simulink model "PlantModelSim"  (R2019b)
settings: Solver=VariableStepAuto  StartTime=0.0  StopTime=10.0  RelTol=1e-3
values from neighbouring files (symbols this model uses):
  A = [0  0  0  1  0  0  0  0  0  0  0  0 ... (first row only)    [Naman_LQR_Working.m]    (also in PlantModel.m = [0  0  0  1  0  0  0  0  0  0  0  0;      0  0  0  0  1  0  )
  B = [0      0       0       0 ... (first row only)    [Naman_LQR_Working.m]    (also in PlantModel.m = [0 0 0 0;      0 0 0 0;      0 0 0 0;      0 0 0 0;      0 0)
  C = [1 0 0 0 0 0 0 0 0 0 0 0 ... (first row only)    [Naman_LQR_Working.m]    (also in PlantModel.m = [1 0 0 0 0 0 0 0 0 0 0 0;      0 1 0 0 0 0 0 0 0 0 0 0;     )
  D = zeros(6,4)    [Naman_LQR_Working.m]    (also in PlantModel.m)
settings Model: Creator=Lakshu  LastModifiedBy=Lakshu

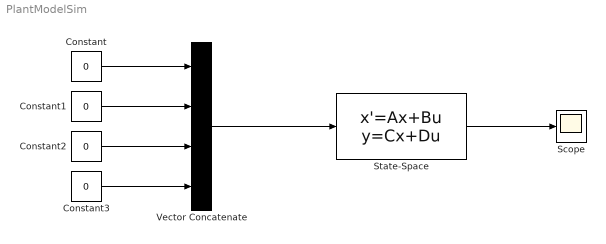
== system PlantModelSim ==
  Constant{,1..3} (4 alike) : Constant  Value=0
  Scope : Scope
  State-Space : StateSpace  A=A  B=B  C=C  D=D  InitialCondition=0
  Vector Concatenate : Concatenate  NumInputs=4
  wires:
  Vector Concatenate/1 -> State-Space/1
  State-Space/1 -> Scope/1
  Constant/1 -> Vector Concatenate/1
  Constant1/1 -> Vector Concatenate/2
  Constant2/1 -> Vector Concatenate/3
  Constant3/1 -> Vector Concatenate/4
